simulink library "xbsReplacements_r2"  (Simulink 5.0)
undefined symbols (not defined in the file or in its folder): N
libraries: xbsReplacements_r2 x122, xbsIO_r2 x35, xbsDSP_r2 x10, xbsComm_r2 x10, xbsMath_r2 x6, xbsBasic_r2 x3, xbsMemory_r2 x1
settings Model: Creator=jballagh  LastModifiedBy=singhj

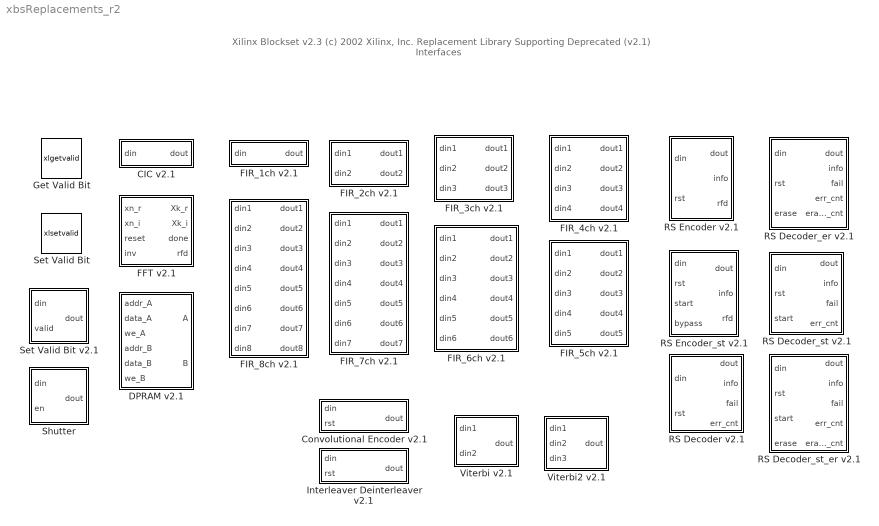
== system xbsReplacements_r2 ==
  note: Xilinx Blockset v2.3
      | (c) 2002 Xilinx, Inc.
      |
      | Replacement Library Supporting
      | Deprecated (v2.1) Interfaces
  CIC v2.1 : Subsystem
      mask Help: web(xldoclink('CIC v2.1'));
  Convolutional Encoder v2.1 : Subsystem
      mask Help: web(xldoclink('Convolutional Encoder v2.1'));
  DPRAM v2.1 : Subsystem
      mask Help: web(xldoclink('DPRAM v2.1'));
  FFT v2.1 : Subsystem
      mask Help: web(xldoclink('FFT v2.1'));
  FIR_1ch v2.1 : Subsystem
      mask Help: web(xldoclink('FIR_1ch v2.1'));
  FIR_2ch v2.1 : Subsystem
      mask Help: web(xldoclink('FIR_2ch v2.1'));
  FIR_3ch v2.1 : Subsystem
      mask Help: web(xldoclink('FIR_3ch v2.1'));
  FIR_4ch v2.1 : Subsystem
      mask Help: web(xldoclink('FIR_4ch v2.1'));
  FIR_5ch v2.1 : Subsystem
      mask Help: web(xldoclink('FIR_5ch v2.1'));
  FIR_6ch v2.1 : Subsystem
      mask Help: web(xldoclink('FIR_6ch v2.1'));
  FIR_7ch v2.1 : Subsystem
      mask Help: web(xldoclink('FIR_7ch v2.1'));
  FIR_8ch v2.1 : Subsystem
      mask Help: web(xldoclink('FIR_8ch v2.1'));
  Get Valid Bit : S-Function  FunctionName=xlgetvalid  Parameters=sfcn_mwsv__  mask(Xilinx Get Valid Bit){}
      mask help: Valid bit extractor. Output is one when input is a valid, and zero otherwise.
      mask init:
      | [designRoot, family, part, speed, package, simulinkPeriod, sysclkPeriod, dbl_ovrd, trimVbit] = xlSysgenSettings(gcb,0,2);
      | [bg,fg] = xlcmap('XBlock');
      | iPos = get_param(gcb,'Position');
      | iWidth=iPos(3)-iPos(1); iHeight=iPos(4)-iPos(2);
      | iCx=iWidth/2;
      | iCy=iHeight/2;
      | [logoX, logoY] = xlogo(iPos);
      | 
      | 
      | % one time added for param list
      | precision0 = 1;
      | dblOvrd = dbl_ovrd;
      | 
      | % just pass everything to s-function
      | sfcn_mwsv__ = get_param(gcb, 'MaskWSVariables');
      mask Help: web(xldoclink('Get Valid Bit'));
      mask Display:
      | patch([0 iWidth iWidth 0],[0 0 iHeight iHeight] , bg);
      | patch(logoX,logoY , fg);
      | port_label('output',1,'valid');
      | 
      | ;plot([0 0 iWidth iWidth 0], [0 iHeight iHeight 0 0]);
  Interleaver Deinterleaver v2.1 : Subsystem
      mask Help: web(xldoclink('Interleaver Deinterleaver v2.1'));
  RS Decoder v2.1 : Subsystem
      mask Help: web(xldoclink('RS Decoder v2.1'));
  RS Decoder_er v2.1 : Subsystem
      mask Help: web(xldoclink('RS Decoder_er v2.1'));
  RS Decoder_st v2.1 : Subsystem
      mask Help: web(xldoclink('RS Decoder_st v2.1'));
  RS Decoder_st_er v2.1 : Subsystem
      mask Help: web(xldoclink('RS Decoder_st_er v2.1'));
  RS Encoder v2.1 : Subsystem
      mask Help: web(xldoclink('RS Encoder v2.1'));
  RS Encoder_st v2.1 : Subsystem
      mask Help: web(xldoclink('RS Encoder_st v2.1'));
  Set Valid Bit : S-Function  FunctionName=xlsetvalid  Parameters=sfcn_mwsv__  mask(Xilinx Set Valid Bit){explicit_period=off, period=1, dbl_ovrd=off}
      mask prompts: explicit_period "Use Explicit Sample Period"; period "Sample Period  (use -1 to inherit first known input period)"; dbl_ovrd "Override with Doubles"
      mask help: Marks samples as valid or invalid. Copies samples from the input to the output, marking each as valid or invalid according to the value presented at the ``valid'' port.
      mask init:
      | [designRoot, family, part, speed, package, simulinkPeriod, sysclkPeriod, dbl_ovrd, trimVbit] = xlSysgenSettings(gcb,1,2);
      | [bg,fg] = xlcmap('XBlock',dbl_ovrd);
      | iPos = get_param(gcb,'Position');
      | iWidth=iPos(3)-iPos(1); iHeight=iPos(4)-iPos(2);
      | iCx=iWidth/2;
      | iCy=iHeight/2;
      | [logoX, logoY] = xlogo(iPos);
      | 
      | 
      | % one time added for param list
      | precision0 = 1;
      | explicitClk = explicit_period;
      | dblOvrd = dbl_ovrd;
      | 
      | % just pass everything to s-function
      | sfcn_mwsv__ = get_param(gcb, 'MaskWSVariables');
      mask Help: web(xldoclink('Set Valid Bit'));
      mask Display:
      | patch([0 iWidth iWidth 0],[0 0 iHeight iHeight] , bg);
      | patch(logoX,logoY , fg);
      | port_label('input',1,'data');
      | port_label('input',2,'valid');
      | 
      | plot([0 0 iWidth iWidth 0], [0 iHeight iHeight 0 0]);
  Set Valid Bit v2.1 : Subsystem
      mask Help: web(xldoclink('Set Valid Bit v2.1'));
  Shutter : Subsystem
      mask Help: web(xldoclink('Shutter'));
  Viterbi v2.1 : Subsystem
      mask Help: web(xldoclink('Viterbi v2.1'));
  Viterbi2 v2.1 : Subsystem
      mask Help: web(xldoclink('Viterbi2 v2.1'));

== system xbsReplacements_r2/CIC v2.1 ==
  din : Inport
  CIC : xbsDSP_r2/CIC  filter_type=Decimator  samp_rate_change=8  stages=2  differential_delay=1  latency=1  explicit_period=off  period=1  dbl_ovrd=off  gen_core=on  use_rpm=on  deprecated_control=on
  Get Valid Bit : xbsReplacements_r2/Get Valid Bit
  Set Valid Bit : xbsReplacements_r2/Set Valid Bit  explicit_period=off  period=1  dbl_ovrd=off
  dout : Outport
  wires:
  Get Valid Bit/1 -> CIC/2
  din/1 -> CIC/1, Get Valid Bit/1
  CIC/2 -> Set Valid Bit/2
  CIC/1 -> Set Valid Bit/1
  Set Valid Bit/1 -> dout/1

== system xbsReplacements_r2/Convolutional Encoder v2.1 ==
  din : Inport
  rst : Inport  Port=2
  Convolutional Encoder : xbsComm_r2/Convolutional Encoder  input_rate=2  output_rate=3  code1_char=[1 1 1]  code2_char=[1 0 1]  code3_char=[1 1 0]  output_type=Single-Channel Output  punctured_code_1='101'  punctured_code_2='101'  explicit_period=off  period=1  rst=on  en=off  dbl_ovrd=off  gen_core=on  use_rpm=on  deprecated_control=on
  Get Valid Bit1 : xbsReplacements_r2/Get Valid Bit
  Set Valid Bit : xbsReplacements_r2/Set Valid Bit  explicit_period=off  period=1  dbl_ovrd=off
  dout : Outport
  wires:
  Get Valid Bit1/1 -> Convolutional Encoder/2
  Set Valid Bit/1 -> dout/1
  Convolutional Encoder/1 -> Set Valid Bit/1
  Convolutional Encoder/2 -> Set Valid Bit/2
  din/1 -> Convolutional Encoder/1, Get Valid Bit1/1
  rst/1 -> Convolutional Encoder/3

== system xbsReplacements_r2/DPRAM v2.1 ==
  addr_A : Inport
  data_A : Inport  Port=2
  we_A : Inport  Port=3
  addr_B : Inport  Port=4
  data_B : Inport  Port=5
  we_B : Inport  Port=6
  Dual Port RAM : xbsMemory_r2/Dual Port RAM  depth=16  initVector=sin(pi*(0:15)/16)  write_mode_A=Read After Write  write_mode_B=Read After Write  latency=1  mem_collision=on  init_zero=on  explicit_period=off  period=1  trim_vbits=off  dbl_ovrd=off  gen_core=on  deprecated_control=on
  Set Valid Bit1 : xbsReplacements_r2/Set Valid Bit  explicit_period=off  period=1  dbl_ovrd=off
  Set Valid Bit3 : xbsReplacements_r2/Set Valid Bit  explicit_period=off  period=1  dbl_ovrd=off
  A : Outport
  B : Outport  Port=2
  wires:
  Set Valid Bit3/1 -> A/1
  Set Valid Bit1/1 -> B/1
  addr_A/1 -> Dual Port RAM/1
  data_A/1 -> Dual Port RAM/2
  we_A/1 -> Dual Port RAM/3
  addr_B/1 -> Dual Port RAM/4
  data_B/1 -> Dual Port RAM/5
  we_B/1 -> Dual Port RAM/6
  Dual Port RAM/1 -> Set Valid Bit3/1
  Dual Port RAM/2 -> Set Valid Bit3/2
  Dual Port RAM/3 -> Set Valid Bit1/1
  Dual Port RAM/4 -> Set Valid Bit1/2

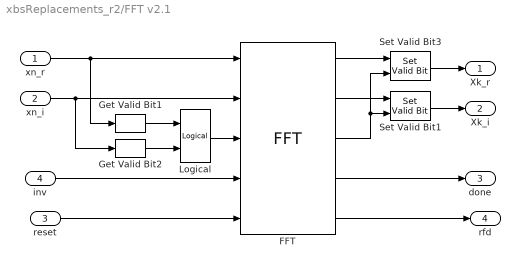
== system xbsReplacements_r2/FFT v2.1 ==
  xn_r : Inport
  xn_i : Inport  Port=2
  reset : Inport  Port=3
  inv : Inport  Port=4
  FFT : xbsDSP_r2/FFT  n=64  mem=Triple  scale_mode=1/N  oflw_inv=on  explicit_period=off  period=1  rst=on  dbl_ovrd=off  gen_core=on  deprecated_control=on
  Get Valid Bit1 : xbsReplacements_r2/Get Valid Bit
  Get Valid Bit2 : xbsReplacements_r2/Get Valid Bit
  Logical : xbsMath_r2/Logical  logical_function=AND  inputs=2  precision=Full  arith_type=Unsigned  n_bits=8  bin_pt=2  align_bp=on  latency=0  explicit_period=off  period=1  en=off  trim_vbits=on  dbl_ovrd=off  use_core=on  gen_core=on  use_rpm=off  deprecated_control=on
  Set Valid Bit1 : xbsReplacements_r2/Set Valid Bit  explicit_period=off  period=1  dbl_ovrd=off
  Set Valid Bit3 : xbsReplacements_r2/Set Valid Bit  explicit_period=off  period=1  dbl_ovrd=off
  Xk_r : Outport
  Xk_i : Outport  Port=2
  done : Outport  Port=3
  rfd : Outport  Port=4
  wires:
  reset/1 -> FFT/5
  inv/1 -> FFT/4
  xn_i/1 -> FFT/2, Get Valid Bit2/1
  xn_r/1 -> FFT/1, Get Valid Bit1/1
  Logical/1 -> FFT/3
  Get Valid Bit1/1 -> Logical/1
  Get Valid Bit2/1 -> Logical/2
  FFT/3 -> Set Valid Bit3/2, Set Valid Bit1/2
  FFT/1 -> Set Valid Bit3/1
  FFT/2 -> Set Valid Bit1/1
  Set Valid Bit1/1 -> Xk_i/1
  Set Valid Bit3/1 -> Xk_r/1
  FFT/4 -> done/1
  FFT/5 -> rfd/1

== system xbsReplacements_r2/FIR_1ch v2.1 ==
  din : Inport
  FIR : xbsDSP_r2/FIR  coef=[1 -1]  structure=Inferred from Coefficients  coef_n_bits=8  coef_bin_pt=6  coef_arith_type="Signed  (2's complement)"  num_channels=1  polyphase_behavior="Single Rate:  sample in - sample out"  latency=1  over_sample=1  explicit_period=off  period=1  dbl_ovrd=off  gen_core=on  deprecated_control=on
  Get Valid Bit : xbsReplacements_r2/Get Valid Bit
  Set Valid Bit : xbsReplacements_r2/Set Valid Bit  explicit_period=off  period=1  dbl_ovrd=off
  dout : Outport
  wires:
  Set Valid Bit/1 -> dout/1
  FIR/1 -> Set Valid Bit/1
  FIR/2 -> Set Valid Bit/2
  din/1 -> Get Valid Bit/1, FIR/1
  Get Valid Bit/1 -> FIR/2

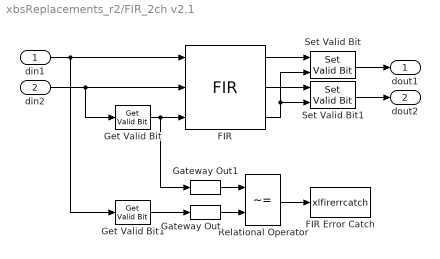
== system xbsReplacements_r2/FIR_2ch v2.1 ==
  din1 : Inport
  din2 : Inport  Port=2
  FIR : xbsDSP_r2/FIR  coef=[1 -1]  structure=Inferred from Coefficients  coef_n_bits=8  coef_bin_pt=6  coef_arith_type="Signed  (2's complement)"  num_channels=2  polyphase_behavior="Single Rate:  sample in - sample out"  latency=1  over_sample=1  explicit_period=off  period=1  dbl_ovrd=off  gen_core=on  deprecated_control=on
  FIR Error Catch : S-Function  FunctionName=xlfirerrcatch
  Gateway Out : xbsIO_r2/Gateway Out  hdl_port=off  timing_constraint=None  locs_specified=off  LOCs={}
  Gateway Out1 : xbsIO_r2/Gateway Out  hdl_port=off  timing_constraint=None  locs_specified=off  LOCs={}
  Get Valid Bit : xbsReplacements_r2/Get Valid Bit
  Get Valid Bit1 : xbsReplacements_r2/Get Valid Bit
  Relational Operator : RelationalOperator  Operator=~=  InputSameDT=on
  Set Valid Bit : xbsReplacements_r2/Set Valid Bit  explicit_period=off  period=1  dbl_ovrd=off
  Set Valid Bit1 : xbsReplacements_r2/Set Valid Bit  explicit_period=off  period=1  dbl_ovrd=off
  dout1 : Outport
  dout2 : Outport  Port=2
  wires:
  Get Valid Bit/1 -> FIR/3, Gateway Out1/1
  Set Valid Bit/1 -> dout1/1
  Set Valid Bit1/1 -> dout2/1
  FIR/1 -> Set Valid Bit/1
  FIR/2 -> Set Valid Bit1/1
  FIR/3 -> Set Valid Bit1/2, Set Valid Bit/2
  din1/1 -> FIR/1, Get Valid Bit1/1
  din2/1 -> FIR/2, Get Valid Bit/1
  Gateway Out1/1 -> Relational Operator/1
  Gateway Out/1 -> Relational Operator/2
  Relational Operator/1 -> FIR Error Catch/1
  Get Valid Bit1/1 -> Gateway Out/1

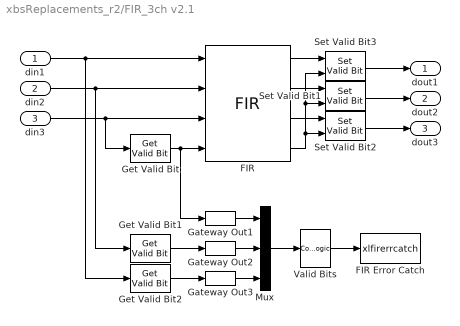
== system xbsReplacements_r2/FIR_3ch v2.1 ==
  din1 : Inport
  din2 : Inport  Port=2
  din3 : Inport  Port=3
  FIR : xbsDSP_r2/FIR  coef=[1 -1]  structure=Inferred from Coefficients  coef_n_bits=8  coef_bin_pt=6  coef_arith_type="Signed  (2's complement)"  num_channels=3  polyphase_behavior="Single Rate:  sample in - sample out"  latency=1  over_sample=1  explicit_period=off  period=1  dbl_ovrd=off  gen_core=on  deprecated_control=on
  FIR Error Catch : S-Function  FunctionName=xlfirerrcatch
  Gateway Out1 : xbsIO_r2/Gateway Out  hdl_port=off  timing_constraint=None  locs_specified=off  LOCs={}
  Gateway Out2 : xbsIO_r2/Gateway Out  hdl_port=off  timing_constraint=None  locs_specified=off  LOCs={}
  Gateway Out3 : xbsIO_r2/Gateway Out  hdl_port=off  timing_constraint=None  locs_specified=off  LOCs={}
  Get Valid Bit : xbsReplacements_r2/Get Valid Bit
  Get Valid Bit1 : xbsReplacements_r2/Get Valid Bit
  Get Valid Bit2 : xbsReplacements_r2/Get Valid Bit
  Mux : Mux  Inputs=3
  Set Valid Bit1 : xbsReplacements_r2/Set Valid Bit  explicit_period=off  period=1  dbl_ovrd=off
  Set Valid Bit2 : xbsReplacements_r2/Set Valid Bit  explicit_period=off  period=1  dbl_ovrd=off
  Set Valid Bit3 : xbsReplacements_r2/Set Valid Bit  explicit_period=off  period=1  dbl_ovrd=off
  Valid Bits : CombinatorialLogic  TruthTable=[0; ones(6,1) ; 0]
  dout1 : Outport
  dout2 : Outport  Port=2
  dout3 : Outport  Port=3
  wires:
  din2/1 -> FIR/2, Get Valid Bit1/1
  din1/1 -> FIR/1, Get Valid Bit2/1
  FIR/2 -> Set Valid Bit1/1
  FIR/1 -> Set Valid Bit3/1
  Set Valid Bit1/1 -> dout2/1
  Set Valid Bit3/1 -> dout1/1
  din3/1 -> FIR/3, Get Valid Bit/1
  Set Valid Bit2/1 -> dout3/1
  FIR/3 -> Set Valid Bit2/1
  FIR/4 -> Set Valid Bit2/2, Set Valid Bit1/2, Set Valid Bit3/2
  Get Valid Bit/1 -> FIR/4, Gateway Out1/1
  Get Valid Bit1/1 -> Gateway Out2/1
  Get Valid Bit2/1 -> Gateway Out3/1
  Gateway Out3/1 -> Mux/3
  Gateway Out2/1 -> Mux/2
  Gateway Out1/1 -> Mux/1
  Mux/1 -> Valid Bits/1
  Valid Bits/1 -> FIR Error Catch/1

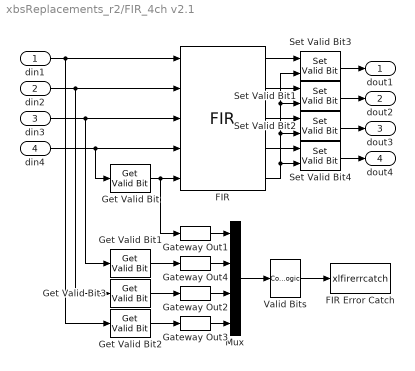
== system xbsReplacements_r2/FIR_4ch v2.1 ==
  din1 : Inport
  din2 : Inport  Port=2
  din3 : Inport  Port=3
  din4 : Inport  Port=4
  FIR : xbsDSP_r2/FIR  coef=[1 -1]  structure=Inferred from Coefficients  coef_n_bits=8  coef_bin_pt=6  coef_arith_type="Signed  (2's complement)"  num_channels=4  polyphase_behavior="Single Rate:  sample in - sample out"  latency=1  over_sample=1  explicit_period=off  period=1  dbl_ovrd=off  gen_core=on  deprecated_control=on
  FIR Error Catch : S-Function  FunctionName=xlfirerrcatch
  Gateway Out{1..4} (4 alike) : xbsIO_r2/Gateway Out  hdl_port=off  timing_constraint=None  locs_specified=off  LOCs={}
  Get Valid Bit{,1..3} (4 alike) : xbsReplacements_r2/Get Valid Bit
  Mux : Mux
  Set Valid Bit{1..4} (4 alike) : xbsReplacements_r2/Set Valid Bit  explicit_period=off  period=1  dbl_ovrd=off
  Valid Bits : CombinatorialLogic  TruthTable=[0; ones(14,1) ;0]
  dout1 : Outport
  dout2 : Outport  Port=2
  dout3 : Outport  Port=3
  dout4 : Outport  Port=4
  wires:
  Valid Bits/1 -> FIR Error Catch/1
  Mux/1 -> Valid Bits/1
  Get Valid Bit2/1 -> Gateway Out3/1
  FIR/3 -> Set Valid Bit2/1
  Set Valid Bit2/1 -> dout3/1
  din3/1 -> FIR/3, Get Valid Bit1/1
  Set Valid Bit3/1 -> dout1/1
  Set Valid Bit1/1 -> dout2/1
  FIR/1 -> Set Valid Bit3/1
  FIR/2 -> Set Valid Bit1/1
  din1/1 -> FIR/1, Get Valid Bit2/1
  din2/1 -> FIR/2, Get Valid Bit3/1
  Set Valid Bit4/1 -> dout4/1
  FIR/4 -> Set Valid Bit4/1
  FIR/5 -> Set Valid Bit4/2, Set Valid Bit2/2, Set Valid Bit1/2, Set Valid Bit3/2
  din4/1 -> FIR/4, Get Valid Bit/1
  Get Valid Bit/1 -> FIR/5, Gateway Out1/1
  Get Valid Bit1/1 -> Gateway Out4/1
  Gateway Out4/1 -> Mux/2
  Gateway Out1/1 -> Mux/1
  Gateway Out2/1 -> Mux/3
  Get Valid Bit3/1 -> Gateway Out2/1
  Gateway Out3/1 -> Mux/4

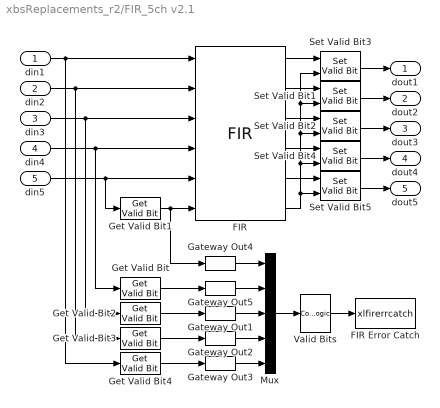
== system xbsReplacements_r2/FIR_5ch v2.1 ==
  din1 : Inport
  din2 : Inport  Port=2
  din3 : Inport  Port=3
  din4 : Inport  Port=4
  din5 : Inport  Port=5
  FIR : xbsDSP_r2/FIR  coef=[1 -1]  structure=Inferred from Coefficients  coef_n_bits=8  coef_bin_pt=6  coef_arith_type="Signed  (2's complement)"  num_channels=5  polyphase_behavior="Single Rate:  sample in - sample out"  latency=1  over_sample=1  explicit_period=off  period=1  dbl_ovrd=off  gen_core=on  deprecated_control=on
  FIR Error Catch : S-Function  FunctionName=xlfirerrcatch
  Gateway Out{1..5} (5 alike) : xbsIO_r2/Gateway Out  hdl_port=off  timing_constraint=None  locs_specified=off  LOCs={}
  Get Valid Bit{,1..4} (5 alike) : xbsReplacements_r2/Get Valid Bit
  Mux : Mux  Inputs=5
  Set Valid Bit{1..5} (5 alike) : xbsReplacements_r2/Set Valid Bit  explicit_period=off  period=1  dbl_ovrd=off
  Valid Bits : CombinatorialLogic  TruthTable=[0; ones(30,1) ; 0]
  dout1 : Outport
  dout2 : Outport  Port=2
  dout3 : Outport  Port=3
  dout4 : Outport  Port=4
  dout5 : Outport  Port=5
  wires:
  din2/1 -> FIR/2, Get Valid Bit3/1
  din1/1 -> FIR/1, Get Valid Bit4/1
  Set Valid Bit1/1 -> dout2/1
  Set Valid Bit3/1 -> dout1/1
  din3/1 -> FIR/3, Get Valid Bit2/1
  Set Valid Bit2/1 -> dout3/1
  Valid Bits/1 -> FIR Error Catch/1
  Set Valid Bit5/1 -> dout5/1
  Set Valid Bit4/1 -> dout4/1
  FIR/5 -> Set Valid Bit5/1
  FIR/4 -> Set Valid Bit4/1
  FIR/3 -> Set Valid Bit2/1
  FIR/2 -> Set Valid Bit1/1
  FIR/1 -> Set Valid Bit3/1
  FIR/6 -> Set Valid Bit5/2, Set Valid Bit4/2, Set Valid Bit2/2, Set Valid Bit1/2, Set Valid Bit3/2
  din4/1 -> FIR/4, Get Valid Bit/1
  din5/1 -> FIR/5, Get Valid Bit1/1
  Get Valid Bit1/1 -> FIR/6, Gateway Out4/1
  Get Valid Bit/1 -> Gateway Out5/1
  Get Valid Bit4/1 -> Gateway Out3/1
  Get Valid Bit3/1 -> Gateway Out2/1
  Get Valid Bit2/1 -> Gateway Out1/1
  Gateway Out3/1 -> Mux/5
  Gateway Out2/1 -> Mux/4
  Gateway Out1/1 -> Mux/3
  Gateway Out5/1 -> Mux/2
  Gateway Out4/1 -> Mux/1
  Mux/1 -> Valid Bits/1

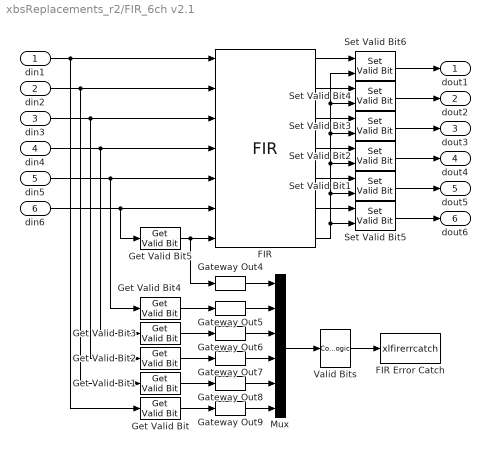
== system xbsReplacements_r2/FIR_6ch v2.1 ==
  din1 : Inport
  din2 : Inport  Port=2
  din3 : Inport  Port=3
  din4 : Inport  Port=4
  din5 : Inport  Port=5
  din6 : Inport  Port=6
  FIR : xbsDSP_r2/FIR  coef=[1 -1]  structure=Inferred from Coefficients  coef_n_bits=8  coef_bin_pt=6  coef_arith_type="Signed  (2's complement)"  num_channels=6  polyphase_behavior="Single Rate:  sample in - sample out"  latency=1  over_sample=1  explicit_period=off  period=1  dbl_ovrd=off  gen_core=on  deprecated_control=on
  FIR Error Catch : S-Function  FunctionName=xlfirerrcatch
  Gateway Out{4..9} (6 alike) : xbsIO_r2/Gateway Out  hdl_port=off  timing_constraint=None  locs_specified=off  LOCs={}
  Get Valid Bit{,1..5} (6 alike) : xbsReplacements_r2/Get Valid Bit
  Mux : Mux  Inputs=6
  Set Valid Bit{1..6} (6 alike) : xbsReplacements_r2/Set Valid Bit  explicit_period=off  period=1  dbl_ovrd=off
  Valid Bits : CombinatorialLogic  TruthTable=[0; ones(62,1) ; 0]
  dout1 : Outport
  dout2 : Outport  Port=2
  dout3 : Outport  Port=3
  dout4 : Outport  Port=4
  dout5 : Outport  Port=5
  dout6 : Outport  Port=6
  wires:
  Valid Bits/1 -> FIR Error Catch/1
  Mux/1 -> Valid Bits/1
  Set Valid Bit3/1 -> dout3/1
  din3/1 -> FIR/3, Get Valid Bit2/1
  Set Valid Bit6/1 -> dout1/1
  Set Valid Bit4/1 -> dout2/1
  din1/1 -> FIR/1, Get Valid Bit/1
  din2/1 -> FIR/2, Get Valid Bit1/1
  FIR/1 -> Set Valid Bit6/1
  FIR/2 -> Set Valid Bit4/1
  FIR/3 -> Set Valid Bit3/1
  FIR/6 -> Set Valid Bit5/1
  FIR/5 -> Set Valid Bit1/1
  FIR/4 -> Set Valid Bit2/1
  Set Valid Bit2/1 -> dout4/1
  Set Valid Bit1/1 -> dout5/1
  Set Valid Bit5/1 -> dout6/1
  din4/1 -> FIR/4, Get Valid Bit3/1
  din5/1 -> FIR/5, Get Valid Bit4/1
  din6/1 -> FIR/6, Get Valid Bit5/1
  Get Valid Bit5/1 -> FIR/7, Gateway Out4/1
  Get Valid Bit/1 -> Gateway Out9/1
  Get Valid Bit1/1 -> Gateway Out8/1
  Get Valid Bit2/1 -> Gateway Out7/1
  Get Valid Bit3/1 -> Gateway Out6/1
  Get Valid Bit4/1 -> Gateway Out5/1
  Gateway Out9/1 -> Mux/6
  Gateway Out8/1 -> Mux/5
  Gateway Out7/1 -> Mux/4
  Gateway Out6/1 -> Mux/3
  Gateway Out5/1 -> Mux/2
  Gateway Out4/1 -> Mux/1
  FIR/7 -> Set Valid Bit5/2, Set Valid Bit1/2, Set Valid Bit2/2, Set Valid Bit3/2, Set Valid Bit4/2, Set Valid Bit6/2

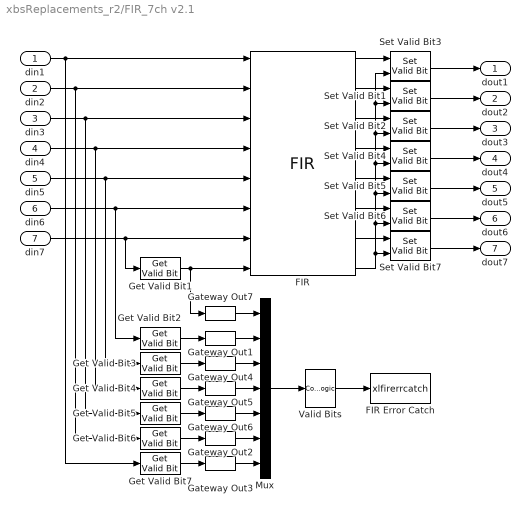
== system xbsReplacements_r2/FIR_7ch v2.1 ==
  din1 : Inport
  din2 : Inport  Port=2
  din3 : Inport  Port=3
  din4 : Inport  Port=4
  din5 : Inport  Port=5
  din6 : Inport  Port=6
  din7 : Inport  Port=7
  FIR : xbsDSP_r2/FIR  coef=[1 -1]  structure=Inferred from Coefficients  coef_n_bits=8  coef_bin_pt=6  coef_arith_type="Signed  (2's complement)"  num_channels=7  polyphase_behavior="Single Rate:  sample in - sample out"  latency=1  over_sample=1  explicit_period=off  period=1  dbl_ovrd=off  gen_core=on  deprecated_control=on
  FIR Error Catch : S-Function  FunctionName=xlfirerrcatch
  Gateway Out{1..7} (7 alike) : xbsIO_r2/Gateway Out  hdl_port=off  timing_constraint=None  locs_specified=off  LOCs={}
  Get Valid Bit{1..7} (7 alike) : xbsReplacements_r2/Get Valid Bit
  Mux : Mux  Inputs=7
  Set Valid Bit{1..7} (7 alike) : xbsReplacements_r2/Set Valid Bit  explicit_period=off  period=1  dbl_ovrd=off
  Valid Bits : CombinatorialLogic  TruthTable=[0; ones(126,1) ; 0]
  dout1 : Outport
  dout2 : Outport  Port=2
  dout3 : Outport  Port=3
  dout4 : Outport  Port=4
  dout5 : Outport  Port=5
  dout6 : Outport  Port=6
  dout7 : Outport  Port=7
  wires:
  din2/1 -> FIR/2, Get Valid Bit6/1
  din1/1 -> FIR/1, Get Valid Bit7/1
  FIR/2 -> Set Valid Bit1/1
  FIR/1 -> Set Valid Bit3/1
  Set Valid Bit1/1 -> dout2/1
  Set Valid Bit3/1 -> dout1/1
  din3/1 -> FIR/3, Get Valid Bit5/1
  Set Valid Bit2/1 -> dout3/1
  FIR/3 -> Set Valid Bit2/1
  Valid Bits/1 -> FIR Error Catch/1
  din4/1 -> FIR/4, Get Valid Bit4/1
  din5/1 -> FIR/5, Get Valid Bit3/1
  din6/1 -> FIR/6, Get Valid Bit2/1
  din7/1 -> FIR/7, Get Valid Bit1/1
  Get Valid Bit1/1 -> FIR/8, Gateway Out7/1
  Set Valid Bit7/1 -> dout7/1
  Set Valid Bit6/1 -> dout6/1
  Set Valid Bit5/1 -> dout5/1
  Set Valid Bit4/1 -> dout4/1
  FIR/4 -> Set Valid Bit4/1
  FIR/5 -> Set Valid Bit5/1
  FIR/6 -> Set Valid Bit6/1
  FIR/7 -> Set Valid Bit7/1
  FIR/8 -> Set Valid Bit7/2, Set Valid Bit6/2, Set Valid Bit5/2, Set Valid Bit4/2, Set Valid Bit2/2, Set Valid Bit1/2, Set Valid Bit3/2
  Get Valid Bit2/1 -> Gateway Out1/1
  Get Valid Bit3/1 -> Gateway Out4/1
  Get Valid Bit4/1 -> Gateway Out5/1
  Get Valid Bit5/1 -> Gateway Out6/1
  Get Valid Bit6/1 -> Gateway Out2/1
  Get Valid Bit7/1 -> Gateway Out3/1
  Gateway Out7/1 -> Mux/1
  Gateway Out1/1 -> Mux/2
  Gateway Out4/1 -> Mux/3
  Gateway Out5/1 -> Mux/4
  Gateway Out6/1 -> Mux/5
  Gateway Out2/1 -> Mux/6
  Gateway Out3/1 -> Mux/7
  Mux/1 -> Valid Bits/1

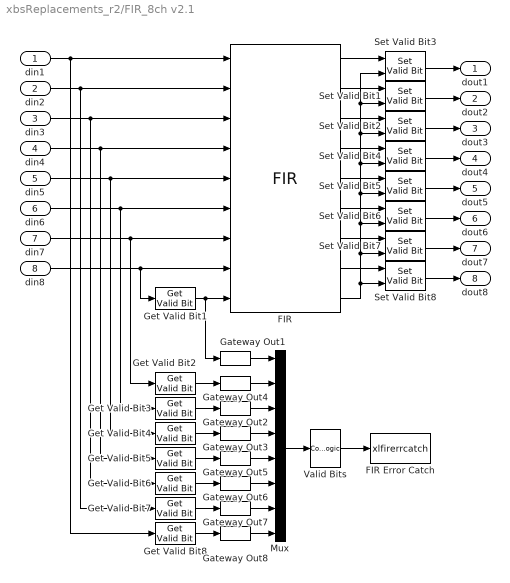
== system xbsReplacements_r2/FIR_8ch v2.1 ==
  din1 : Inport
  din2 : Inport  Port=2
  din3 : Inport  Port=3
  din4 : Inport  Port=4
  din5 : Inport  Port=5
  din6 : Inport  Port=6
  din7 : Inport  Port=7
  din8 : Inport  Port=8
  FIR : xbsDSP_r2/FIR  coef=[1 -1]  structure=Inferred from Coefficients  coef_n_bits=8  coef_bin_pt=6  coef_arith_type="Signed  (2's complement)"  num_channels=8  polyphase_behavior="Single Rate:  sample in - sample out"  latency=1  over_sample=1  explicit_period=off  period=1  valids=on  dbl_ovrd=off  gen_core=on  deprecated_control=on
  FIR Error Catch : S-Function  FunctionName=xlfirerrcatch
  Gateway Out{1..8} (8 alike) : xbsIO_r2/Gateway Out  hdl_port=off  timing_constraint=None  locs_specified=off  LOCs={}
  Get Valid Bit{1..8} (8 alike) : xbsReplacements_r2/Get Valid Bit
  Mux : Mux  Inputs=8
  Set Valid Bit{1..8} (8 alike) : xbsReplacements_r2/Set Valid Bit  explicit_period=off  period=1  dbl_ovrd=off
  Valid Bits : CombinatorialLogic  TruthTable=[0; ones(254,1) ;0]
  dout1 : Outport
  dout2 : Outport  Port=2
  dout3 : Outport  Port=3
  dout4 : Outport  Port=4
  dout5 : Outport  Port=5
  dout6 : Outport  Port=6
  dout7 : Outport  Port=7
  dout8 : Outport  Port=8
  wires:
  Valid Bits/1 -> FIR Error Catch/1
  Set Valid Bit2/1 -> dout3/1
  din3/1 -> FIR/3, Get Valid Bit6/1
  Set Valid Bit3/1 -> dout1/1
  Set Valid Bit1/1 -> dout2/1
  din1/1 -> FIR/1, Get Valid Bit8/1
  din2/1 -> FIR/2, Get Valid Bit7/1
  Get Valid Bit1/1 -> FIR/9, Gateway Out1/1
  din4/1 -> FIR/4, Get Valid Bit5/1
  din5/1 -> FIR/5, Get Valid Bit4/1
  din6/1 -> FIR/6, Get Valid Bit3/1
  din7/1 -> FIR/7, Get Valid Bit2/1
  din8/1 -> FIR/8, Get Valid Bit1/1
  FIR/4 -> Set Valid Bit4/1
  FIR/3 -> Set Valid Bit2/1
  FIR/2 -> Set Valid Bit1/1
  FIR/1 -> Set Valid Bit3/1
  FIR/8 -> Set Valid Bit8/1
  FIR/7 -> Set Valid Bit7/1
  FIR/6 -> Set Valid Bit6/1
  FIR/5 -> Set Valid Bit5/1
  FIR/9 -> Set Valid Bit8/2, Set Valid Bit7/2, Set Valid Bit6/2, Set Valid Bit5/2, Set Valid Bit4/2, Set Valid Bit2/2, Set Valid Bit1/2, Set Valid Bit3/2
  Set Valid Bit8/1 -> dout8/1
  Set Valid Bit7/1 -> dout7/1
  Set Valid Bit6/1 -> dout6/1
  Set Valid Bit5/1 -> dout5/1
  Set Valid Bit4/1 -> dout4/1
  Get Valid Bit2/1 -> Gateway Out4/1
  Get Valid Bit8/1 -> Gateway Out8/1
  Get Valid Bit7/1 -> Gateway Out7/1
  Get Valid Bit6/1 -> Gateway Out6/1
  Get Valid Bit5/1 -> Gateway Out5/1
  Get Valid Bit4/1 -> Gateway Out3/1
  Get Valid Bit3/1 -> Gateway Out2/1
  Gateway Out1/1 -> Mux/1
  Gateway Out4/1 -> Mux/2
  Gateway Out2/1 -> Mux/3
  Gateway Out3/1 -> Mux/4
  Gateway Out5/1 -> Mux/5
  Gateway Out6/1 -> Mux/6
  Gateway Out7/1 -> Mux/7
  Gateway Out8/1 -> Mux/8
  Mux/1 -> Valid Bits/1

== system xbsReplacements_r2/Interleaver Deinterleaver v2.1 ==
  din : Inport
  rst : Inport  Port=2
  Get Valid Bit1 : xbsReplacements_r2/Get Valid Bit
  Interleaver Deinterleaver : xbsComm_r2/Interleaver Deinterleaver  mode=Interleaver  num_branches=3  branch_length=[2 4 5]  mem_type=Automatically Chosen  pipeline=off  explicit_period=off  period=1  rst=on  en=off  dbl_ovrd=off  gen_core=on  use_rpm=on  deprecated_control=on
  Set Valid Bit1 : xbsReplacements_r2/Set Valid Bit  explicit_period=off  period=1  dbl_ovrd=off
  dout : Outport
  wires:
  Interleaver Deinterleaver/2 -> Set Valid Bit1/2
  Interleaver Deinterleaver/1 -> Set Valid Bit1/1
  Set Valid Bit1/1 -> dout/1
  Get Valid Bit1/1 -> Interleaver Deinterleaver/2
  din/1 -> Interleaver Deinterleaver/1, Get Valid Bit1/1
  rst/1 -> Interleaver Deinterleaver/3

== system xbsReplacements_r2/RS Decoder v2.1 ==
  din : Inport
  rst : Inport  Port=2
  Get Valid Bit1 : xbsReplacements_r2/Get Valid Bit
  RS Decoder : xbsComm_r2/RS Decoder  code_spec=Custom  sym_width=8  nn=204  kk=188  poly_char=[ 1 0 0 0 1 1 1 0 1]  gen_start=0  scale=1  hasStart=off  hasErase=off  explicit_period=off  period=1  rst=on  dbl_ovrd=off  gen_core=on  use_rpm=on  deprecated_control=on
  Set Valid Bit{1..4} (4 alike) : xbsReplacements_r2/Set Valid Bit  explicit_period=off  period=1  dbl_ovrd=off
  dout : Outport
  info : Outport  Port=2
  fail : Outport  Port=3
  err_cnt : Outport  Port=4
  wires:
  Get Valid Bit1/1 -> RS Decoder/2
  rst/1 -> RS Decoder/3
  Set Valid Bit1/1 -> dout/1
  din/1 -> RS Decoder/1, Get Valid Bit1/1
  RS Decoder/1 -> Set Valid Bit1/1
  Set Valid Bit2/1 -> info/1
  RS Decoder/3 -> Set Valid Bit2/1
  Set Valid Bit3/1 -> fail/1
  Set Valid Bit4/1 -> err_cnt/1
  RS Decoder/4 -> Set Valid Bit3/1
  RS Decoder/5 -> Set Valid Bit4/1
  RS Decoder/2 -> Set Valid Bit4/2, Set Valid Bit3/2, Set Valid Bit2/2, Set Valid Bit1/2

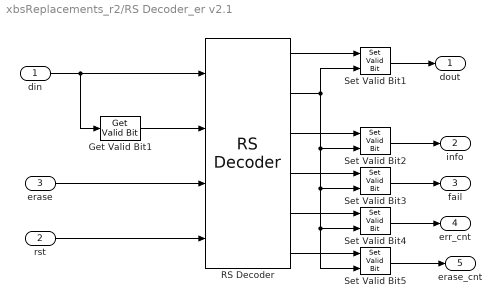
== system xbsReplacements_r2/RS Decoder_er v2.1 ==
  din : Inport
  rst : Inport  Port=2
  erase : Inport  Port=3
  Get Valid Bit1 : xbsReplacements_r2/Get Valid Bit
  RS Decoder : xbsComm_r2/RS Decoder  code_spec=Custom  sym_width=8  nn=204  kk=188  poly_char=[ 1 0 0 0 1 1 1 0 1]  gen_start=0  scale=1  hasStart=off  hasErase=on  explicit_period=off  period=1  rst=on  dbl_ovrd=off  gen_core=on  use_rpm=on  deprecated_control=on
  Set Valid Bit{1..5} (5 alike) : xbsReplacements_r2/Set Valid Bit  explicit_period=off  period=1  dbl_ovrd=off
  dout : Outport
  info : Outport  Port=2
  fail : Outport  Port=3
  err_cnt : Outport  Port=4
  erase_cnt : Outport  Port=5
  wires:
  erase/1 -> RS Decoder/3
  rst/1 -> RS Decoder/4
  Get Valid Bit1/1 -> RS Decoder/2
  Set Valid Bit1/1 -> dout/1
  din/1 -> RS Decoder/1, Get Valid Bit1/1
  RS Decoder/1 -> Set Valid Bit1/1
  Set Valid Bit2/1 -> info/1
  RS Decoder/3 -> Set Valid Bit2/1
  Set Valid Bit3/1 -> fail/1
  Set Valid Bit4/1 -> err_cnt/1
  RS Decoder/4 -> Set Valid Bit3/1
  RS Decoder/5 -> Set Valid Bit4/1
  RS Decoder/2 -> Set Valid Bit3/2, Set Valid Bit4/2, Set Valid Bit5/2, Set Valid Bit2/2, Set Valid Bit1/2
  RS Decoder/6 -> Set Valid Bit5/1
  Set Valid Bit5/1 -> erase_cnt/1

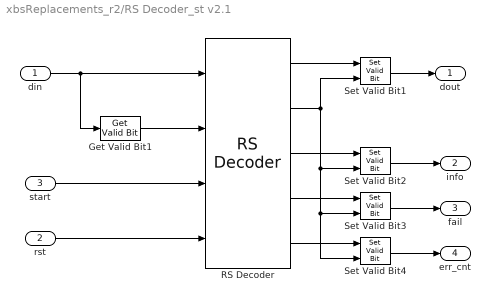
== system xbsReplacements_r2/RS Decoder_st v2.1 ==
  din : Inport
  rst : Inport  Port=2
  start : Inport  Port=3
  Get Valid Bit1 : xbsReplacements_r2/Get Valid Bit
  RS Decoder : xbsComm_r2/RS Decoder  code_spec=Custom  sym_width=8  nn=204  kk=188  poly_char=[ 1 0 0 0 1 1 1 0 1]  gen_start=0  scale=1  hasStart=on  hasErase=off  explicit_period=off  period=1  rst=on  dbl_ovrd=off  gen_core=on  use_rpm=on  deprecated_control=on
  Set Valid Bit{1..4} (4 alike) : xbsReplacements_r2/Set Valid Bit  explicit_period=off  period=1  dbl_ovrd=off
  dout : Outport
  info : Outport  Port=2
  fail : Outport  Port=3
  err_cnt : Outport  Port=4
  wires:
  RS Decoder/2 -> Set Valid Bit1/2, Set Valid Bit2/2, Set Valid Bit3/2, Set Valid Bit4/2
  RS Decoder/5 -> Set Valid Bit4/1
  RS Decoder/4 -> Set Valid Bit3/1
  Set Valid Bit4/1 -> err_cnt/1
  Set Valid Bit3/1 -> fail/1
  RS Decoder/3 -> Set Valid Bit2/1
  Set Valid Bit2/1 -> info/1
  RS Decoder/1 -> Set Valid Bit1/1
  din/1 -> Get Valid Bit1/1, RS Decoder/1
  Set Valid Bit1/1 -> dout/1
  Get Valid Bit1/1 -> RS Decoder/2
  rst/1 -> RS Decoder/4
  start/1 -> RS Decoder/3

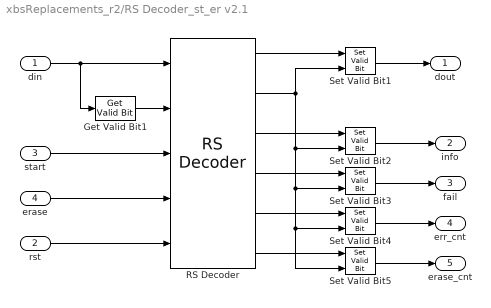
== system xbsReplacements_r2/RS Decoder_st_er v2.1 ==
  din : Inport
  rst : Inport  Port=2
  start : Inport  Port=3
  erase : Inport  Port=4
  Get Valid Bit1 : xbsReplacements_r2/Get Valid Bit
  RS Decoder : xbsComm_r2/RS Decoder  code_spec=Custom  sym_width=8  nn=204  kk=188  poly_char=[ 1 0 0 0 1 1 1 0 1]  gen_start=0  scale=1  hasStart=on  hasErase=on  explicit_period=off  period=1  rst=on  dbl_ovrd=off  gen_core=on  use_rpm=on  deprecated_control=on
  Set Valid Bit{1..5} (5 alike) : xbsReplacements_r2/Set Valid Bit  explicit_period=off  period=1  dbl_ovrd=off
  dout : Outport
  info : Outport  Port=2
  fail : Outport  Port=3
  err_cnt : Outport  Port=4
  erase_cnt : Outport  Port=5
  wires:
  start/1 -> RS Decoder/3
  erase/1 -> RS Decoder/4
  Get Valid Bit1/1 -> RS Decoder/2
  Set Valid Bit1/1 -> dout/1
  din/1 -> RS Decoder/1, Get Valid Bit1/1
  RS Decoder/1 -> Set Valid Bit1/1
  Set Valid Bit2/1 -> info/1
  RS Decoder/3 -> Set Valid Bit2/1
  Set Valid Bit3/1 -> fail/1
  Set Valid Bit4/1 -> err_cnt/1
  RS Decoder/4 -> Set Valid Bit3/1
  RS Decoder/5 -> Set Valid Bit4/1
  RS Decoder/2 -> Set Valid Bit3/2, Set Valid Bit4/2, Set Valid Bit5/2, Set Valid Bit2/2, Set Valid Bit1/2
  RS Decoder/6 -> Set Valid Bit5/1
  Set Valid Bit5/1 -> erase_cnt/1
  rst/1 -> RS Decoder/5

== system xbsReplacements_r2/RS Encoder v2.1 ==
  din : Inport
  rst : Inport  Port=2
  Get Valid Bit1 : xbsReplacements_r2/Get Valid Bit
  RS Encoder : xbsComm_r2/RS Encoder  code_spec=Custom  sym_width=8  nn=204  kk=188  poly_char=[ 1 0 0 0 1 1 1 0 1]  gen_start=0  scale=1  hasStart=off  explicit_period=off  period=1  rst=on  dbl_ovrd=off  gen_core=on  use_rpm=on  deprecated_control=on
  Set Valid Bit1 : xbsReplacements_r2/Set Valid Bit  explicit_period=off  period=1  dbl_ovrd=off
  Set Valid Bit2 : xbsReplacements_r2/Set Valid Bit  explicit_period=off  period=1  dbl_ovrd=off
  dout : Outport
  info : Outport  Port=2
  rfd : Outport  Port=3
  wires:
  din/1 -> Get Valid Bit1/1, RS Encoder/1
  Set Valid Bit1/1 -> dout/1
  rst/1 -> RS Encoder/3
  Get Valid Bit1/1 -> RS Encoder/2
  RS Encoder/1 -> Set Valid Bit1/1
  RS Encoder/2 -> Set Valid Bit1/2, Set Valid Bit2/2
  RS Encoder/4 -> rfd/1
  Set Valid Bit2/1 -> info/1
  RS Encoder/3 -> Set Valid Bit2/1

== system xbsReplacements_r2/RS Encoder_st v2.1 ==
  din : Inport
  rst : Inport  Port=2
  start : Inport  Port=3
  bypass : Inport  Port=4
  Get Valid Bit1 : xbsReplacements_r2/Get Valid Bit
  RS Encoder : xbsComm_r2/RS Encoder  code_spec=Custom  sym_width=8  nn=204  kk=188  poly_char=[ 1 0 0 0 1 1 1 0 1]  gen_start=0  scale=1  hasStart=on  explicit_period=off  period=1  rst=on  dbl_ovrd=off  gen_core=on  use_rpm=on  deprecated_control=on
  Set Valid Bit1 : xbsReplacements_r2/Set Valid Bit  explicit_period=off  period=1  dbl_ovrd=off
  Set Valid Bit2 : xbsReplacements_r2/Set Valid Bit  explicit_period=off  period=1  dbl_ovrd=off
  dout : Outport
  info : Outport  Port=2
  rfd : Outport  Port=3
  wires:
  RS Encoder/3 -> Set Valid Bit2/1
  Set Valid Bit2/1 -> info/1
  RS Encoder/4 -> rfd/1
  RS Encoder/2 -> Set Valid Bit2/2, Set Valid Bit1/2
  RS Encoder/1 -> Set Valid Bit1/1
  Set Valid Bit1/1 -> dout/1
  din/1 -> RS Encoder/1, Get Valid Bit1/1
  Get Valid Bit1/1 -> RS Encoder/2
  start/1 -> RS Encoder/3
  bypass/1 -> RS Encoder/4
  rst/1 -> RS Encoder/5

== system xbsReplacements_r2/Set Valid Bit v2.1 ==
  note: din_valid   valid    valid_valid
      | 0         0           0
      | 0         0           1
      | 0         1           0
      | 0         1           1
      | 1         0           0
      | 1         0           1
      | 1         1           0
      | 1         1           1
  note: dout_valid
      | 0
      | 0
      | 0
      | 0
      | 1
      | 0
      | 1
      | 1
  note: <--- In version 2.1, the "Set Valid Bit" block only
      |      changed the valid bit for dout in the case where
      |      din was valid and the "valid" port input was
      |      zero and marked as valid).
  note: Truth Table:
  note: This subsystem reproduces the behavior supplied by the Set Valid Bit block in v2.1 of the Xilinx Blockset.
  din : Inport
  valid : Inport  Port=2
  Convert : xbsBasic_r2/Convert  arith_type=Boolean  n_bits=1  bin_pt=0  quantization=Truncate  overflow=Wrap  latency=0  explicit_period=off  period=1  trim_vbits=on  dbl_ovrd=off  inserted_by_tool=off  deprecated_control=off
  Get Valid Bit : xbsReplacements_r2/Get Valid Bit
  Get Valid Bit1 : xbsReplacements_r2/Get Valid Bit
  Inverter : xbsMath_r2/Inverter  latency=0  explicit_period=off  period=1  en=off  trim_vbits=on  dbl_ovrd=off  use_core=off  gen_core=on  use_rpm=off  deprecated_control=off
  Logical : xbsMath_r2/Logical  logical_function=AND  inputs=2  precision=Full  arith_type=Unsigned  n_bits=8  bin_pt=2  align_bp=off  latency=0  explicit_period=off  period=1  en=off  trim_vbits=off  dbl_ovrd=off  use_core=off  gen_core=on  use_rpm=off  deprecated_control=on
  Logical1 : xbsMath_r2/Logical  logical_function=OR  inputs=2  precision=Full  arith_type=Unsigned  n_bits=8  bin_pt=2  align_bp=off  latency=0  explicit_period=off  period=1  en=off  trim_vbits=off  dbl_ovrd=off  use_core=off  gen_core=on  use_rpm=off  deprecated_control=on
  Set Valid Bit : xbsReplacements_r2/Set Valid Bit  explicit_period=off  period=1  dbl_ovrd=off
  dout : Outport
  wires:
  valid/1 -> Get Valid Bit1/1, Convert/1
  Get Valid Bit/1 -> Logical/1
  Logical/1 -> Set Valid Bit/2
  din/1 -> Get Valid Bit/1, Set Valid Bit/1
  Set Valid Bit/1 -> dout/1
  Get Valid Bit1/1 -> Inverter/1
  Logical1/1 -> Logical/2
  Convert/1 -> Logical1/2
  Inverter/1 -> Logical1/1

== system xbsReplacements_r2/Shutter ==
  din : Inport
  en : Inport  Port=2
  Mux : xbsBasic_r2/Mux  inputs=2  precision=Full  arith_type="Signed  (2's comp)"  n_bits=8  bin_pt=2  quantization=Truncate  overflow=Wrap  latency=0  mux_type=off  explicit_period=off  period=1  en=off  trim_vbits=on  dbl_ovrd=off  gen_core=on  use_rpm=off  deprecated_control=off
      settings: xl_area=[0, 0, 0, 0, 0, 0, 0]
  Register1 : xbsBasic_r2/Register  init=0  reg_only_valid=off  explicit_period=off  period=1  rst=off  en=on  out_en=off  trim_vbits=on  dbl_ovrd=off  deprecated_control=off
      settings: xl_area=[0, 0, 0, 0, 0, 0, 0]
  dout : Outport
  wires:
  din/1 -> Mux/3, Register1/1
  Register1/1 -> Mux/2
  Mux/1 -> dout/1
  en/1 -> Mux/1, Register1/2

== system xbsReplacements_r2/Viterbi v2.1 ==
  din1 : Inport
  din2 : Inport  Port=2
  Get Valid Bit1 : xbsReplacements_r2/Get Valid Bit
  Get Valid Bit2 : xbsReplacements_r2/Get Valid Bit
  Logical : xbsMath_r2/Logical  logical_function=AND  inputs=2  precision=Full  arith_type=Unsigned  n_bits=8  bin_pt=2  align_bp=on  latency=0  explicit_period=off  period=1  en=off  trim_vbits=off  dbl_ovrd=off  use_core=off  gen_core=on  use_rpm=off  deprecated_control=on
  Set Valid Bit1 : xbsReplacements_r2/Set Valid Bit  explicit_period=off  period=1  dbl_ovrd=off
  Viterbi Decoder : xbsComm_r2/Viterbi Decoder  input_rate=2  output_rate=2  tb_length=15  code1_char=[ 1 1 1]  code2_char=[1 0 1]  code3_char=[1 1 0]  punctured_code_1='10'  punctured_code_2='11'  coding=Hard  data_format=Signed Magnitude  explicit_period=off  period=1  dbl_ovrd=off  gen_core=on  use_rpm=on  deprecated_control=on
  dout : Outport
  wires:
  din1/1 -> Viterbi Decoder/1, Get Valid Bit1/1
  din2/1 -> Viterbi Decoder/2, Get Valid Bit2/1
  Viterbi Decoder/1 -> Set Valid Bit1/1
  Viterbi Decoder/2 -> Set Valid Bit1/2
  Set Valid Bit1/1 -> dout/1
  Get Valid Bit2/1 -> Logical/2
  Get Valid Bit1/1 -> Logical/1
  Logical/1 -> Viterbi Decoder/3

== system xbsReplacements_r2/Viterbi2 v2.1 ==
  din1 : Inport
  din2 : Inport  Port=2
  din3 : Inport  Port=3
  Get Valid Bit1 : xbsReplacements_r2/Get Valid Bit
  Get Valid Bit2 : xbsReplacements_r2/Get Valid Bit
  Get Valid Bit3 : xbsReplacements_r2/Get Valid Bit
  Logical : xbsMath_r2/Logical  logical_function=AND  inputs=3  precision=Full  arith_type=Unsigned  n_bits=8  bin_pt=2  align_bp=on  latency=0  explicit_period=off  period=1  en=off  trim_vbits=off  dbl_ovrd=off  use_core=off  gen_core=on  use_rpm=off  deprecated_control=on
  Set Valid Bit1 : xbsReplacements_r2/Set Valid Bit  explicit_period=off  period=1  dbl_ovrd=off
  Viterbi Decoder : xbsComm_r2/Viterbi Decoder  input_rate=2  output_rate=3  tb_length=15  code1_char=[ 1 1 1]  code2_char=[1 0 1]  code3_char=[1 1 0]  punctured_code_1='10'  punctured_code_2='11'  coding=Hard  data_format=Signed Magnitude  explicit_period=off  period=1  gen_core=on  use_rpm=on  deprecated_control=on
  dout : Outport
  wires:
  din1/1 -> Viterbi Decoder/1, Get Valid Bit1/1
  din2/1 -> Viterbi Decoder/2, Get Valid Bit2/1
  din3/1 -> Viterbi Decoder/3, Get Valid Bit3/1
  Viterbi Decoder/1 -> Set Valid Bit1/1
  Viterbi Decoder/2 -> Set Valid Bit1/2
  Set Valid Bit1/1 -> dout/1
  Get Valid Bit3/1 -> Logical/3
  Get Valid Bit2/1 -> Logical/2
  Get Valid Bit1/1 -> Logical/1
  Logical/1 -> Viterbi Decoder/4
